simulink model "math"  (Simulink 7.3)
settings: Solver=FixedStepDiscrete  StartTime=0.0  StopTime=10.0  FixedStep=1  RelTol=1e-3
undefined symbols (not defined in the file): magnitude
settings Model: Creator=ksmyth  LastModifiedBy=hnine
settings OptimizationCC: InitFltsAndDblsToZero=on
settings DebuggingCC: SaveWithParameterizedLinksMsg=none
settings GRTTargetCC: TargetFcnLib=ansi_tfl_tmw.mat

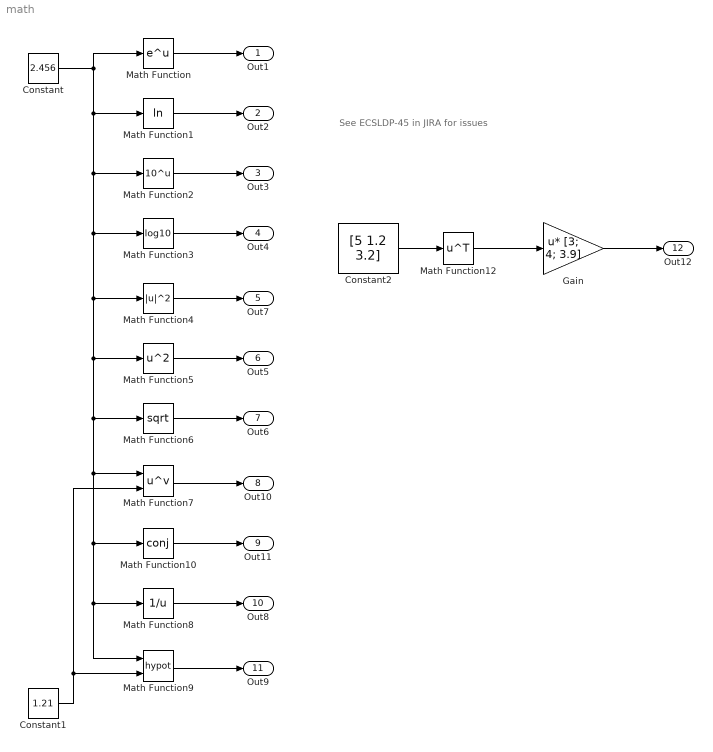
== system math ==
  note: See ECSLDP-45 in JIRA for issues
  Constant : Constant  Value=2.456  OutDataType=sfix(16)  OutScaling=2^0
  Constant1 : Constant  Value=1.21  OutDataType=sfix(16)  OutScaling=2^0
  Constant2 : Constant  Value=[5 1.2 3.2]  OutDataType=sfix(16)  OutScaling=2^0
  Gain : Gain  Gain=[3; 4; 3.9]  Multiplication=Matrix(u*K)  ParameterDataType=sfix(16)  ParameterScaling=2^0  OutDataType=sfix(16)  OutScaling=2^0
  Math Function : Math  OutDataType=sfix(16)  OutScaling=2^0  SaturateOnIntegerOverflow=on
  Math Function1 : Math  Operator=log  OutDataType=sfix(16)  OutScaling=2^0  SaturateOnIntegerOverflow=on
  Math Function10 : Math  Operator=conj  OutDataType=sfix(16)  OutScaling=2^0  SaturateOnIntegerOverflow=on
  Math Function12 : Math  Operator=transpose  OutDataType=sfix(16)  OutScaling=2^0  SaturateOnIntegerOverflow=on
  Math Function2 : Math  Operator=10^u  OutDataType=sfix(16)  OutScaling=2^0  SaturateOnIntegerOverflow=on
  Math Function3 : Math  Operator=log10  OutDataType=sfix(16)  OutScaling=2^0  SaturateOnIntegerOverflow=on
  Math Function4 : Math  Operator=magnitude^2  OutDataType=sfix(16)  OutScaling=2^0  SaturateOnIntegerOverflow=on
  Math Function5 : Math  Operator=square  OutDataType=sfix(16)  OutScaling=2^0  SaturateOnIntegerOverflow=on
  Math Function6 : Math  Operator=sqrt  OutDataType=sfix(16)  OutScaling=2^0  SaturateOnIntegerOverflow=on
  Math Function7 : Math  Operator=pow  OutDataType=sfix(16)  OutScaling=2^0  SaturateOnIntegerOverflow=on
  Math Function8 : Math  Operator=reciprocal  OutDataType=sfix(16)  OutScaling=2^0  SaturateOnIntegerOverflow=on
  Math Function9 : Math  Operator=hypot  OutDataType=sfix(16)  OutScaling=2^0  SaturateOnIntegerOverflow=on
  Out1 : Outport  OutDataType=sfix(16)  OutScaling=2^0
  Out2 : Outport  Port=2  OutDataType=sfix(16)  OutScaling=2^0
  Out3 : Outport  Port=3  OutDataType=sfix(16)  OutScaling=2^0
  Out4 : Outport  Port=4  OutDataType=sfix(16)  OutScaling=2^0
  Out7 : Outport  Port=5  OutDataType=sfix(16)  OutScaling=2^0
  Out5 : Outport  Port=6  OutDataType=sfix(16)  OutScaling=2^0
  Out6 : Outport  Port=7  OutDataType=sfix(16)  OutScaling=2^0
  Out10 : Outport  Port=8  OutDataType=sfix(16)  OutScaling=2^0
  Out11 : Outport  Port=9  OutDataType=sfix(16)  OutScaling=2^0
  Out8 : Outport  Port=10  OutDataType=sfix(16)  OutScaling=2^0
  Out9 : Outport  Port=11  OutDataType=sfix(16)  OutScaling=2^0
  Out12 : Outport  Port=12  OutDataType=sfix(16)  OutScaling=2^0
  wires:
  Constant/1 -> Math Function/1, Math Function3/1, Math Function6/1, Math Function7/1, Math Function8/1, Math Function9/1, Math Function10/1, Math Function5/1, Math Function4/1, Math Function2/1, Math Function1/1
  Math Function/1 -> Out1/1
  Math Function1/1 -> Out2/1
  Math Function2/1 -> Out3/1
  Math Function3/1 -> Out4/1
  Math Function5/1 -> Out5/1
  Math Function6/1 -> Out6/1
  Math Function8/1 -> Out8/1
  Constant1/1 -> Math Function7/2, Math Function9/2
  Math Function9/1 -> Out9/1
  Constant2/1 -> Math Function12/1
  Math Function12/1 -> Gain/1
  Gain/1 -> Out12/1
  Math Function4/1 -> Out7/1
  Math Function7/1 -> Out10/1
  Math Function10/1 -> Out11/1
